simulink model "Mod5Counter"  (R2020a)
settings: Solver=VariableStepAuto  StartTime=0.0  StopTime=10.0  RelTol=1e-3
settings Model: Creator=DELL  LastModifiedBy=DELL

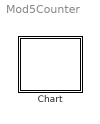
== system Mod5Counter ==
  Chart : Stateflow chart  TreatAsAtomicUnit=on

== stateflow chart Mod5Counter/Chart ==
  state State1
    entry:
    x=0;
    y=0;
    z=0;
    c=0;
  state State5
    entry:
    x=1;
    y=0;
    z=0;
    c=5;
  state State2
    entry:
    x=0;
    y=0;
    z=1;
    c=1;
  state State4
    entry:
    x=0;
    y=1;
    z=1;
    c=4;
  state State3
    entry:
    x=0;
    y=1;
    z=0;
    c=3;
  (default) -> State1
  State5 -> State1 : {x==1&&y==0&&z==0}
  State1 -> State2 : {x==0&&y==0&&z==0}
  State4 -> State5 : {x==0&&y==1&&z==1}
  State2 -> State3 : {x==0&&y==0&&z==1}
  State3 -> State4 : {x==0&&y==1&&z==0}
